simulink model "main_luenberger"  (R2016b)
settings: Solver=ode45  StartTime=0.0  StopTime=200  FixedStep=Par.Step_size  RelTol=1e-3
undefined symbols (not defined in the file or in its folder): now, Par
settings Model: Creator=Ørjan  LastModifiedBy=Ørjan
settings DataIOCC: InitialState=init  SaveState=on  ReturnWorkspaceOutputs=on  ReturnWorkspaceOutputsName=spidata
settings RTWCC: RTWCompilerOptimization=on
settings CodeAppCC: MaxIdLength=95

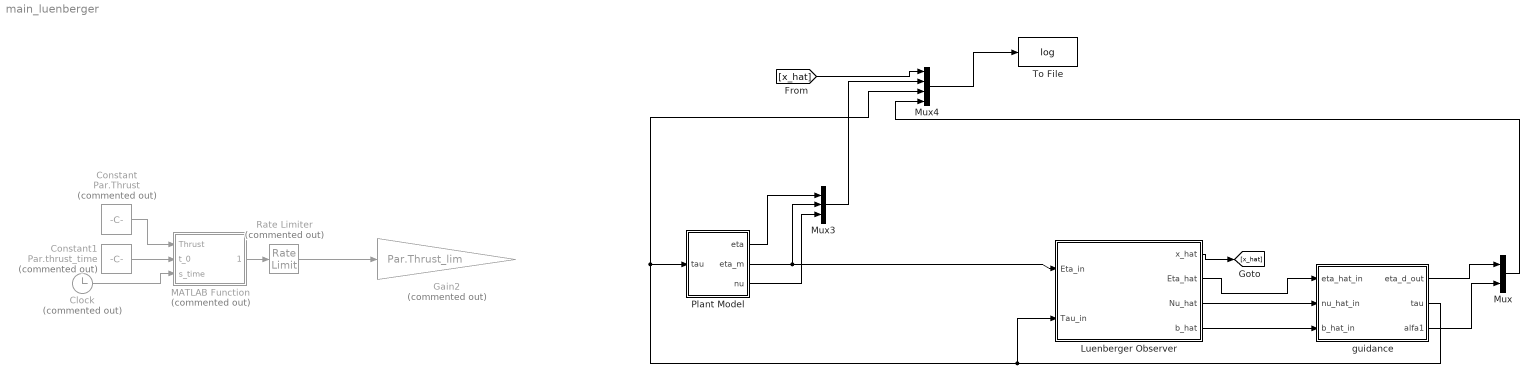
== system main_luenberger ==
  Clock : Clock  Commented=on
  Constant : Constant  Commented=on  Value=Par.Thrust  VectorParams1D=off
  Constant1 : Constant  Commented=on  Value=Par.thrust_time
  Gain2 : Gain  Commented=on  Gain=Par.Thrust_lim
  Luenberger Observer : Subsystem
  MATLAB Function : MATLAB Function  Commented=on  TreatAsAtomicUnit=on
  Mux : Mux  Inputs=2
  Mux3 : Mux  Inputs=3
  Mux4 : Mux
  Plant Model : Subsystem
  Rate Limiter : RateLimiter  Commented=on  RisingSlewLimit=5  FallingSlewLimit=-5  SampleTimeMode=inherited
  To File : ToFile  Filename=log  MatrixName=x  SampleTime=0.1
  guidance : Subsystem
  wires:
  Constant/1 -> MATLAB Function/1(Thrust)
  Clock/1 -> MATLAB Function/3(s_time)
  MATLAB Function/1(tau_norm) -> Rate Limiter/1
  Constant1/1 -> MATLAB Function/2(t_0)
  guidance/2(tau) -> Mux4/3, Plant Model/1(tau), Luenberger Observer/2(Tau_in)
  Rate Limiter/1 -> Gain2/1
  Plant Model/2(eta_m) -> Mux3/2, Luenberger Observer/1(Eta_in)
  Plant Model/1(eta) -> Mux3/1
  Plant Model/3(nu) -> Mux3/3
  Mux3/1 -> Mux4/2
  Mux4/1 -> To File/1
  [x_hat] -> Mux4/1
  Luenberger Observer/1("x_hat ") -> [x_hat]
  Luenberger Observer/3(Nu_hat) -> guidance/2(nu_hat_in)
  Luenberger Observer/2(Eta_hat) -> guidance/1("eta_hat_in ")
  Mux/1 -> Mux4/4
  Luenberger Observer/4(b_hat) -> guidance/3(b_hat_in)
  guidance/3(alfa1) -> Mux/2
  guidance/1(eta_d_out) -> Mux/1

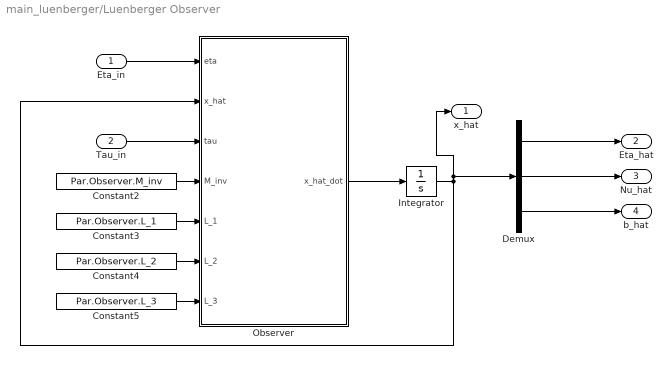
== system main_luenberger/Luenberger Observer ==
  Eta_in : Inport
  Tau_in : Inport  Port=2
  Constant2 : Constant  Value=Par.Observer.M_inv
  Constant3 : Constant  Value=Par.Observer.L_1
  Constant4 : Constant  Value=Par.Observer.L_2
  Constant5 : Constant  Value=Par.Observer.L_3
  Demux : Demux  Outputs=3
  Integrator : Integrator  InitialCondition=Par.Observer.x_0
  Observer : MATLAB Function  TreatAsAtomicUnit=on
  "x_hat " : Outport
  Eta_hat : Outport  Port=2  PortDimensions=[3, 1]
  Nu_hat : Outport  Port=3  PortDimensions=[3, 1]
  b_hat : Outport  Port=4  PortDimensions=[3, 1]
  wires:
  Constant3/1 -> Observer/5(L_1)
  Integrator/1 -> "x_hat "/1, Demux/1, Observer/2(x_hat)
  Demux/1 -> Eta_hat/1
  Demux/2 -> Nu_hat/1
  Observer/1(x_hat_dot) -> Integrator/1
  Constant2/1 -> Observer/4(M_inv)
  Eta_in/1 -> Observer/1(eta)
  Tau_in/1 -> Observer/3(tau)
  Constant4/1 -> Observer/6(L_2)
  Constant5/1 -> Observer/7(L_3)
  Demux/3 -> b_hat/1

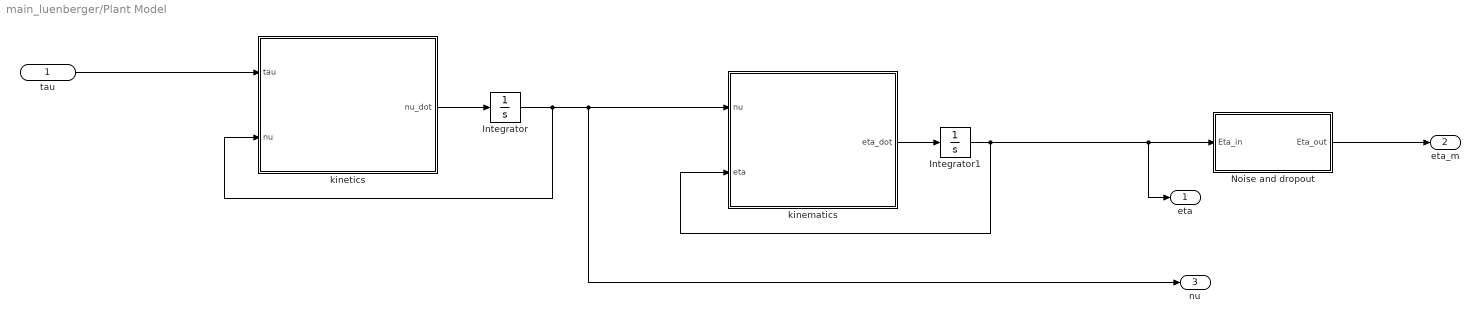
== system main_luenberger/Plant Model ==
  tau : Inport
  Integrator : Integrator  InitialCondition=[0 0 0]
  Integrator1 : Integrator  InitialCondition=[0 0 0]
  Noise and dropout : Subsystem
  kinematics : MATLAB Function  TreatAsAtomicUnit=on
  kinetics : MATLAB Function  TreatAsAtomicUnit=on
  eta : Outport
  eta_m : Outport  Port=2
  nu : Outport  Port=3
  wires:
  kinetics/1(nu_dot) -> Integrator/1
  kinematics/1(eta_dot) -> Integrator1/1
  Integrator/1 -> kinetics/2(nu), nu/1, kinematics/1(nu)
  Integrator1/1 -> eta/1, Noise and dropout/1(Eta_in), kinematics/2(eta)
  Noise and dropout/1(Eta_out) -> eta_m/1
  tau/1 -> kinetics/1(tau)

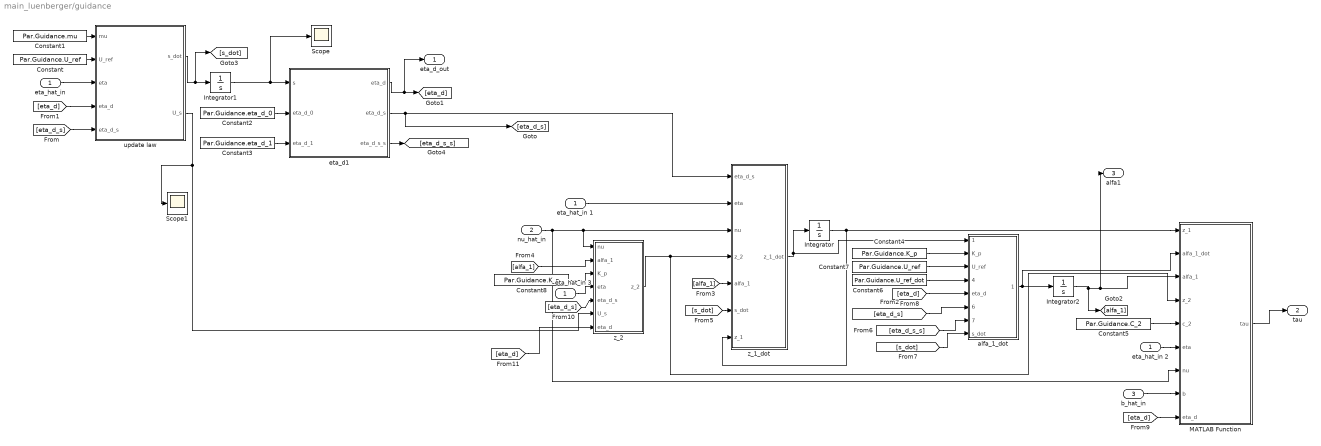
== system main_luenberger/guidance ==
  "eta_hat_in " : Inport
  nu_hat_in : Inport  Port=2
  b_hat_in : Inport  Port=3
  Constant : Constant  Value=Par.Guidance.U_ref
  Constant1 : Constant  Value=Par.Guidance.mu
  Constant2 : Constant  Value=Par.Guidance.eta_d_0
  Constant3 : Constant  Value=Par.Guidance.eta_d_1
  Constant4 : Constant  Value=Par.Guidance.K_p
  Constant5 : Constant  Value=Par.Guidance.C_2
  Constant6 : Constant  Value=Par.Guidance.U_ref_dot
  Constant7 : Constant  Value=Par.Guidance.U_ref
  Constant8 : Constant  Value=Par.Guidance.K_p
  Integrator : Integrator  InitialCondition=Par.Guidance.z_1_0
  Integrator1 : Integrator  InitialCondition=Par.Guidance.s_0
  Integrator2 : Integrator  InitialCondition=Par.Guidance.alfa_1_0
  MATLAB Function : MATLAB Function  TreatAsAtomicUnit=on
  Scope : Scope
  Scope1 : Scope
  alfa_1_dot : MATLAB Function  TreatAsAtomicUnit=on
  eta_d1 : MATLAB Function  TreatAsAtomicUnit=on
  eta_hat_in 1 : InportShadow
  eta_hat_in 2 : InportShadow
  eta_hat_in 3 : InportShadow
  update law : MATLAB Function  TreatAsAtomicUnit=on
  z_1_dot : MATLAB Function  TreatAsAtomicUnit=on
  z_2 : MATLAB Function  TreatAsAtomicUnit=on
  eta_d_out : Outport
  tau : Outport  Port=2
  alfa1 : Outport  Port=3
  wires:
  "eta_hat_in "/1 -> update law/3(eta)
  Constant/1 -> update law/2(U_ref)
  Constant1/1 -> update law/1(mu)
  update law/1(s_dot) -> [s_dot], Integrator1/1
  Integrator1/1 -> Scope/1, eta_d1/1(s)
  Constant2/1 -> eta_d1/2(eta_d_0)
  Constant3/1 -> eta_d1/3(eta_d_1)
  eta_d1/2(eta_d_s) -> [eta_d_s], z_1_dot/1(eta_d_s)
  [eta_d_s] -> update law/5(eta_d_s)
  eta_d1/1(eta_d) -> eta_d_out/1, [eta_d]
  [eta_d] -> update law/4(eta_d)
  nu_hat_in/1 -> z_2/1(nu), z_1_dot/3(nu), MATLAB Function/7(nu)
  eta_hat_in 1/1 -> z_1_dot/2(eta)
  z_1_dot/1(z_1_dot) -> Integrator/1, alfa_1_dot/1(z_1_dot)
  z_2/1(z_2) -> MATLAB Function/4(z_2), z_1_dot/4(z_2)
  Constant4/1 -> alfa_1_dot/2(K_p)
  [eta_d_s] -> alfa_1_dot/6(eta_d_s)
  alfa_1_dot/1(alfa_1_dot) -> MATLAB Function/2(alfa_1_dot), Integrator2/1
  Integrator/1 -> z_1_dot/7(z_1), MATLAB Function/1(z_1)
  Constant5/1 -> MATLAB Function/5(c_2)
  MATLAB Function/1(tau) -> tau/1
  Constant6/1 -> alfa_1_dot/4(U_ref_dot)
  Integrator2/1 -> alfa1/1, MATLAB Function/3(alfa_1), [alfa_1]
  [alfa_1] -> z_1_dot/5(alfa_1)
  [alfa_1] -> z_2/2(alfa_1)
  [s_dot] -> z_1_dot/6(s_dot)
  update law/2(U_s) -> z_2/6(U_s), Scope1/1
  b_hat_in/1 -> MATLAB Function/8(b)
  eta_hat_in 2/1 -> MATLAB Function/6(eta)
  [eta_d_s_s] -> alfa_1_dot/7(eta_d_s_s)
  [s_dot] -> alfa_1_dot/8(s_dot)
  eta_d1/3(eta_d_s_s) -> [eta_d_s_s]
  [eta_d] -> alfa_1_dot/5(eta_d)
  Constant7/1 -> alfa_1_dot/3(U_ref)
  [eta_d] -> MATLAB Function/9(eta_d)
  Constant8/1 -> z_2/3(K_p)
  eta_hat_in 3/1 -> z_2/4(eta)
  [eta_d_s] -> z_2/5(eta_d_s)
  [eta_d] -> z_2/7(eta_d)

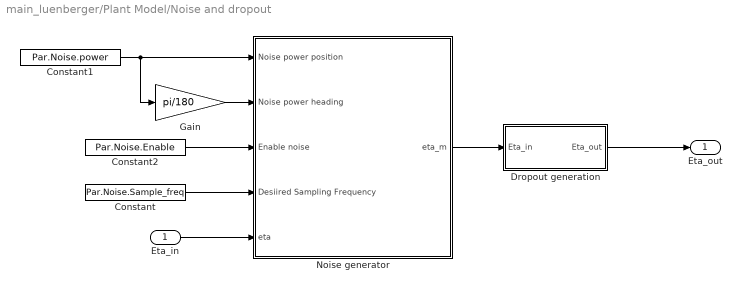
== system main_luenberger/Plant Model/Noise and dropout ==
  Eta_in : Inport
  Constant : Constant  Value=Par.Noise.Sample_freq
  Constant1 : Constant  Value=Par.Noise.power
  Constant2 : Constant  Value=Par.Noise.Enable
  Dropout generation : Subsystem
  Gain : Gain  Gain=pi/180
  Noise generator : Subsystem
  Eta_out : Outport
  wires:
  Constant2/1 -> Noise generator/3(Enable noise)
  Constant/1 -> Noise generator/4(Desiired Sampling Frequency)
  Gain/1 -> Noise generator/2(Noise power heading)
  Constant1/1 -> Noise generator/1(Noise power position), Gain/1
  Eta_in/1 -> Noise generator/5(eta)
  Noise generator/1(eta_m) -> Dropout generation/1(Eta_in)
  Dropout generation/1(Eta_out) -> Eta_out/1

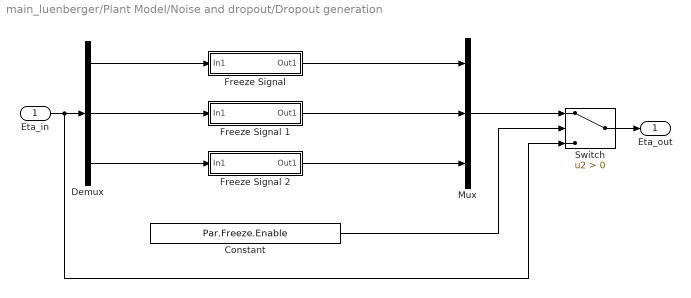
== system main_luenberger/Plant Model/Noise and dropout/Dropout generation ==
  Eta_in : Inport
  Constant : Constant  Value=Par.Freeze.Enable
  Demux : Demux  Outputs=3
  "Freeze Signal " : Subsystem
  Freeze Signal 1 : Subsystem
  Freeze Signal 2 : Subsystem
  Mux : Mux  Inputs=3
  Switch : Switch  Criteria=u2 > Threshold
  Eta_out : Outport
  wires:
  Switch/1 -> Eta_out/1
  Constant/1 -> Switch/2
  Freeze Signal 2/1(Out1) -> Mux/3
  Demux/3 -> Freeze Signal 2/1(In1)
  Demux/2 -> Freeze Signal 1/1(In1)
  Freeze Signal 1/1(Out1) -> Mux/2
  "Freeze Signal "/1(Out1) -> Mux/1
  Demux/1 -> "Freeze Signal "/1(In1)
  Mux/1 -> Switch/1
  Eta_in/1 -> Demux/1, Switch/3

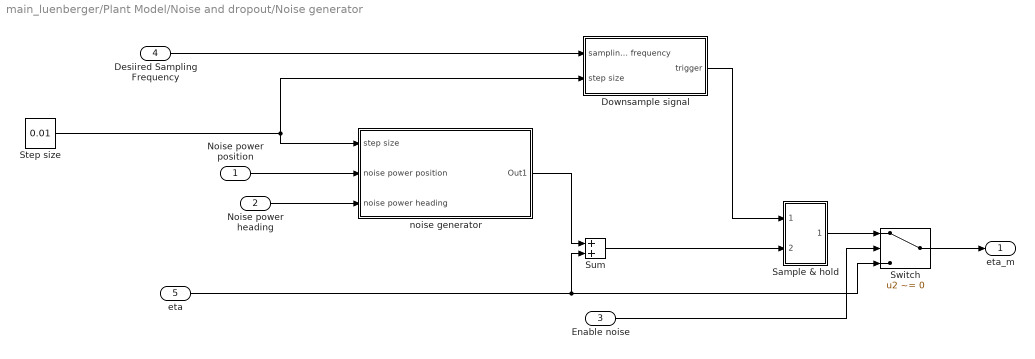
== system main_luenberger/Plant Model/Noise and dropout/Noise generator ==
  Noise power position : Inport
  Noise power heading : Inport  Port=2
  Enable noise : Inport  Port=3
  Desiired Sampling Frequency : Inport  Port=4
  eta : Inport  Port=5
  Downsample	signal : Subsystem
  Sample & hold : Subsystem
  Step size : Constant  Value=0.01
  Sum : Sum
  Switch : Switch  Criteria=u2 ~= 0
  noise generator : Subsystem
  eta_m : Outport
  wires:
  Switch/1 -> eta_m/1
  Enable noise/1 -> Switch/2
  noise generator/1(Out1) -> Sum/1
  Noise power heading/1 -> noise generator/3(noise power heading)
  Noise power position/1 -> noise generator/2(noise power position)
  Sample & hold/1(output) -> Switch/1
  Sum/1 -> Sample & hold/2(input)
  eta/1 -> Switch/3, Sum/2
  Desiired Sampling Frequency/1 -> Downsample	signal/1(sampling frequency)
  Downsample	signal/1(trigger) -> Sample & hold/1(trigger)
  Step size/1 -> noise generator/1(step size), Downsample	signal/2(step size)

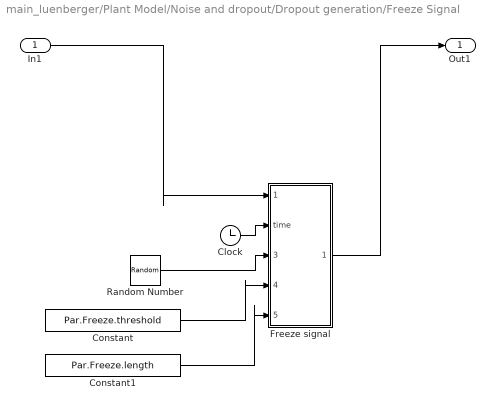
== system main_luenberger/Plant Model/Noise and dropout/Dropout generation/Freeze Signal  ==
  In1 : Inport
  Clock : Clock
  Constant : Constant  Value=Par.Freeze.threshold
  Constant1 : Constant  Value=Par.Freeze.length
  Freeze signal : MATLAB Function  TreatAsAtomicUnit=on
  Random Number : RandomNumber  Seed=ceil(abs(5*round(abs(now*1e6 - fix(now*1e6))*1e5)))  SampleTime=Par.Sample_time
  Out1 : Outport
  wires:
  Random Number/1 -> Freeze signal/3(random_value)
  Clock/1 -> Freeze signal/2(time)
  Constant/1 -> Freeze signal/4(threshold)
  Freeze signal/1(eta_out) -> Out1/1
  In1/1 -> Freeze signal/1(eta_in)
  Constant1/1 -> Freeze signal/5(length)

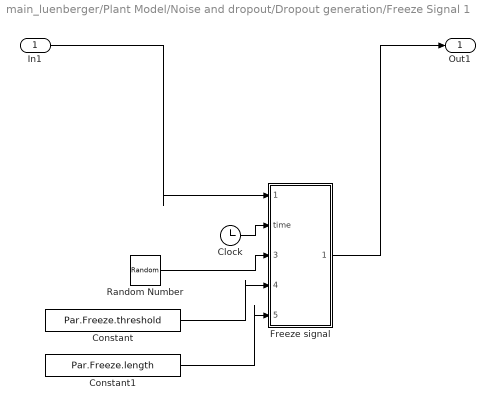
== system main_luenberger/Plant Model/Noise and dropout/Dropout generation/Freeze Signal 1 ==
  In1 : Inport
  Clock : Clock
  Constant : Constant  Value=Par.Freeze.threshold
  Constant1 : Constant  Value=Par.Freeze.length
  Freeze signal : MATLAB Function  TreatAsAtomicUnit=on
  Random Number : RandomNumber  Seed=ceil(abs(5*round(abs(now*1e6 - fix(now*1e6))*1e5)))  SampleTime=Par.Sample_time
  Out1 : Outport
  wires:
  Random Number/1 -> Freeze signal/3(random_value)
  Clock/1 -> Freeze signal/2(time)
  Constant/1 -> Freeze signal/4(threshold)
  Freeze signal/1(eta_out) -> Out1/1
  In1/1 -> Freeze signal/1(eta_in)
  Constant1/1 -> Freeze signal/5(length)

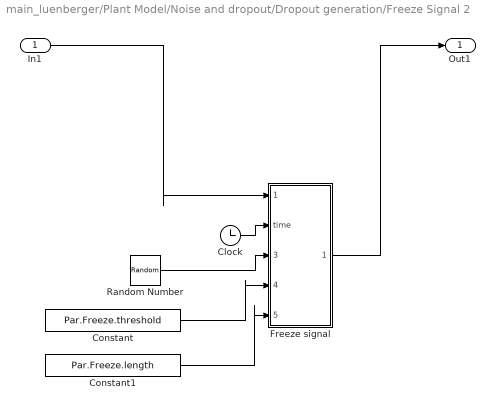
== system main_luenberger/Plant Model/Noise and dropout/Dropout generation/Freeze Signal 2 ==
  In1 : Inport
  Clock : Clock
  Constant : Constant  Value=Par.Freeze.threshold
  Constant1 : Constant  Value=Par.Freeze.length
  Freeze signal : MATLAB Function  TreatAsAtomicUnit=on
  Random Number : RandomNumber  Seed=ceil(abs(5*round(abs(now*1e6 - fix(now*1e6))*1e5)))  SampleTime=Par.Sample_time
  Out1 : Outport
  wires:
  Random Number/1 -> Freeze signal/3(random_value)
  Clock/1 -> Freeze signal/2(time)
  Constant/1 -> Freeze signal/4(threshold)
  Freeze signal/1(eta_out) -> Out1/1
  In1/1 -> Freeze signal/1(eta_in)
  Constant1/1 -> Freeze signal/5(length)

== system main_luenberger/Plant Model/Noise and dropout/Noise generator/Downsample	signal ==
  sampling frequency : Inport
  step size : Inport  Port=2
  MATLAB Function : MATLAB Function  TreatAsAtomicUnit=on
  counter : Memory
  trigger : Outport
  wires:
  MATLAB Function/1(count) -> trigger/1, counter/1
  counter/1 -> MATLAB Function/3(i)
  step size/1 -> MATLAB Function/2(h)
  sampling frequency/1 -> MATLAB Function/1(f)

== system main_luenberger/Plant Model/Noise and dropout/Noise generator/Sample & hold ==
  trigger : Inport
  input : Inport  Port=2
  Hold : Memory
  MATLAB Function1 : MATLAB Function  TreatAsAtomicUnit=on
  output : Outport
  wires:
  Hold/1 -> MATLAB Function1/3(hold)
  input/1 -> MATLAB Function1/2(input)
  trigger/1 -> MATLAB Function1/1(counter)
  MATLAB Function1/1(output) -> Hold/1, output/1

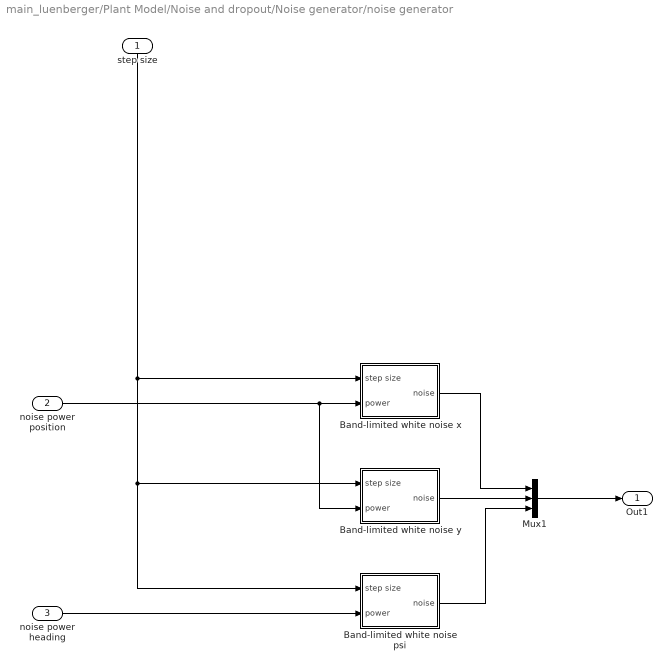
== system main_luenberger/Plant Model/Noise and dropout/Noise generator/noise generator ==
  step size : Inport
  noise power position : Inport  Port=2
  noise power heading : Inport  Port=3
  Band-limited white noise psi : Subsystem
  Band-limited white noise x : Subsystem
  Band-limited white noise y : Subsystem
  Mux1 : Mux  Inputs=3
  Out1 : Outport
  wires:
  noise power heading/1 -> Band-limited white noise psi/2(power)
  Band-limited white noise psi/1(noise) -> Mux1/3
  Band-limited white noise y/1(noise) -> Mux1/2
  Band-limited white noise x/1(noise) -> Mux1/1
  noise power position/1 -> Band-limited white noise x/2(power), Band-limited white noise y/2(power)
  step size/1 -> Band-limited white noise y/1(step size), Band-limited white noise psi/1(step size), Band-limited white noise x/1(step size)
  Mux1/1 -> Out1/1

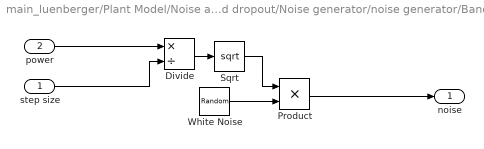
== system main_luenberger/Plant Model/Noise and dropout/Noise generator/noise generator/Band-limited white noise psi ==
  step size : Inport
  power : Inport  Port=2
  Divide : Product  Inputs=*/
  Product : Product
  Sqrt : Sqrt  SaturateOnIntegerOverflow=on
  White Noise : RandomNumber  DisableCoverage=on  Seed=9025  SampleTime=Par.Sample_time
  noise : Outport
  wires:
  power/1 -> Divide/1
  Sqrt/1 -> Product/1
  Divide/1 -> Sqrt/1
  step size/1 -> Divide/2
  Product/1 -> noise/1
  White Noise/1 -> Product/2

== system main_luenberger/Plant Model/Noise and dropout/Noise generator/noise generator/Band-limited white noise x ==
  step size : Inport
  power : Inport  Port=2
  Divide : Product  Inputs=*/
  Product : Product
  Sqrt : Sqrt  SaturateOnIntegerOverflow=on
  White Noise : RandomNumber  DisableCoverage=on  Seed=9024  SampleTime=Par.Sample_time
  noise : Outport
  wires:
  power/1 -> Divide/1
  Sqrt/1 -> Product/1
  Divide/1 -> Sqrt/1
  step size/1 -> Divide/2
  Product/1 -> noise/1
  White Noise/1 -> Product/2

== system main_luenberger/Plant Model/Noise and dropout/Noise generator/noise generator/Band-limited white noise y ==
  step size : Inport
  power : Inport  Port=2
  Divide : Product  Inputs=*/
  Product : Product
  Sqrt : Sqrt  SaturateOnIntegerOverflow=on
  White Noise : RandomNumber  DisableCoverage=on  Seed=123  SampleTime=Par.Sample_time
  noise : Outport
  wires:
  power/1 -> Divide/1
  Sqrt/1 -> Product/1
  Divide/1 -> Sqrt/1
  step size/1 -> Divide/2
  Product/1 -> noise/1
  White Noise/1 -> Product/2

== matlab function main_luenberger/Plant Model/kinematics ==
  data: nu input; eta_dot output; eta input
function eta_dot = CSE1_eta_dot(nu,eta)

psi = eta(3);

J = [cos(psi) -sin(psi) 0
     sin(psi) cos(psi)  0
     0        0         1];

eta_dot = J*nu;

== matlab function main_luenberger/Plant Model/kinetics ==
  data: tau input; nu_dot output; nu input
function nu_dot = CSE1_nu_dot(tau,nu)

u   = nu(1);
v   = nu(2);
r   = nu(3);

tau = [tau(1);tau(2);tau(3)];
%% MATRICES

m    = 14.79;   I_z  =  1.7600;   x_g = 0.0375;       % x_g  =  0.0460; % Table B.1


%% Added mass
X_ud  =     -2.0;											% Table B.1
					Y_vd =     -1.0;	N_vd =    -0.0;		% Table B.1 guestimate
					Y_rd =      -0.0;	N_rd =    -1.0;		% Table B.1

%% Total mass matrix
m_11 = m-X_ud;
m_22 = m-Y_vd;
m_23 = m*x_g-Y_rd;
m_32 = m*x_g-N_vd;
m_33 = I_z-N_rd;

M    = [m_11 0    0
        0    m_22 m_23
        0    m_32 m_33];
	
%% Damping coefficients
% Comments at the end of the lines indicate the old values used.
X_u		= -0.6555;		X_v		= 0;
X_uu 	= 0.3545;		X_vv	= -2.443;
X_uuu 	= -3.787;		X_vvv	= 0;

						Y_v		= -1.33; 			Y_r		= -7.250; % Y_r
						Y_vv	= -2.776;			Y_rr	= -3.450; % Y_rr
						Y_vvv	= -64.91;			Y_rrr	= 0;
						
						Y_rv	= -0.805;			Y_vr	= -0.845; % Y_rv, Y_vr

						N_v		= 0;				N_r		= -1.900; % N_r
						N_vv	= -0.2088;			N_rr	= -0.750; % N_rr
						N_vvv	= 0;				N_rrr	= 0;
						
						N_rv	= 0.130;			N_vr	= 0.080; % N_rv, N_vr

%% Correolis matrix
c_13 = -(m-Y_vd)*v-(m*x_g-Y_rd)*r;
c_23 = (m-X_ud)*u;
C    = [0     0     c_13
        0     0     c_23
        -c_13 -c_23 0   ];

%% Assembly of the damping matrix
d_11 = -X_u - X_uu*u - X_uuu*u^2;
d_22 = -Y_v - Y_vv*v - Y_vvv*v^2 - Y_rv*abs(r);
d_33 = -N_r - N_rr*abs(r) - N_rrr*r^2 - N_vr*abs(v); % using abs(r)

d_12 = -X_v - X_vv*v - X_vvv*v^2;
d_23 = -Y_r - Y_rr*abs(r) - Y_rrr*r^2 - Y_vr*abs(v);
d_32 = -N_v - N_vv*v - N_vvv*v^2 - N_rv*abs(r);

D    = [d_11 d_12 0
        0    d_22 d_23
        0    d_32 d_33];



%% CALCULATION
nu_dot = M\(tau-(C+D)*nu);

== matlab function main_luenberger/guidance/eta_d1 ==
  data: eta_d output size=3; s input; eta_d_0 input; eta_d_1 input; eta_d_s output; eta_d_s_s output
function [eta_d, eta_d_s, eta_d_s_s] = eta_d(s, eta_d_0, eta_d_1)
%% eta_d
x_d = (eta_d_1(1) - eta_d_0(1))*s + eta_d_0(1);
y_d = (eta_d_1(2) - eta_d_0(2))*s + eta_d_0(2);
psi_d = atan(y_d/x_d);
eta_d = [x_d; y_d; psi_d];

%% eta_d_s
x_d_s = eta_d_1(1) - eta_d_0(1);
y_d_s = eta_d_1(2) - eta_d_0(2);
psi_d_s = (y_d_s*eta_d(1) - eta_d(2)*x_d_s)/(eta_d(1)^2 + eta_d(2)^2);
eta_d_s = [x_d_s;y_d_s; psi_d_s];

%% eta_d_s_s
x_d_s_s = 0;
y_d_s_s = 0;
psi_d_s_s = (-2*(y_d_s*x_d - y_d*x_d_s)*(x_d*x_d_s + y_d*y_d_s))/(x_d^2+y_d^2)^2;
eta_d_s_s = [x_d_s_s;y_d_s_s;psi_d_s_s];
end

== matlab function main_luenberger/MATLAB Function ==
  data: tau_norm output; Thrust input; t_0 input; s_time input
function tau_norm = fcn(Thrust, t_0, s_time)
%coder.extrinsic('get_param');
tau_norm = zeros(3,1);
persistent i;
persistent tau;
if(isempty(i))
    i = 1;
end
if(isempty(tau))
    tau = [0; 0; 0];
end
if(s_time>t_0(i))
    tau(1) = Thrust(i, 1);
    tau(2) = Thrust(i, 2);
    tau(3) = Thrust(i, 3);
    if(i<size(Thrust, 1))
        i = i +1;
    end
end
tau_norm = tau;
end

== matlab function main_luenberger/guidance/update law ==
  data: mu input; s_dot output size=1; U_ref input; eta input; eta_d input; eta_d_s input; U_s output
function [s_dot, U_s] = s_dot(mu, U_ref, eta, eta_d, eta_d_s)
psi = eta(3);

R = [cos(psi) -sin(psi) 0; sin(psi) cos(psi) 0; 0 0 1];
z = R'*(eta-eta_d);
U_s = abs(U_ref)/norm(eta_d_s(1:2), 2);
V_1_s = -z'*R'*eta_d_s;
V_1_s = -(eta-eta_d)'*eta_d_s;
s_dot = U_s - (mu/norm(eta_d_s, 2))*V_1_s;
end

== matlab function main_luenberger/guidance/z_1_dot ==
  data: eta_d_s input; eta input; nu input; z_2 input; z_1_dot output size=3; alfa_1 input; s_dot input; z_1 input
function z_1_dot = z_1_dot(eta_d_s, eta, nu, z_2, alfa_1, s_dot, z_1)
psi = eta(3);
r = nu(3);
R = [cos(psi) -sin(psi) 0; sin(psi) cos(psi) 0; 0 0 1];
S = [0 -r 0; r 0 0; 0 0 0];
% z_1_dot = -S*z_1 + z_2 + alfa_1 - R'*eta_d_s*s_dot;
z_1_dot = -S*z_1 + nu - R'*eta_d_s*s_dot;
end

== matlab function main_luenberger/guidance/z_2 ==
  data: nu input; z_2 output; alfa_1 input size=3; K_p input; eta input; eta_d_s input; U_s input; eta_d input
function z_2= z_2(nu, alfa_1, K_p, eta, eta_d_s, U_s, eta_d)
psi = eta(3);
R = [cos(psi), -sin(psi), 0; sin(psi), cos(psi), 0; 0 0 1];
z_1 = R'*(eta-eta_d);
alfa1 = -K_p*z_1 + eta_d_s*U_s;
z_2 = nu - alfa_1;
end

== matlab function main_luenberger/guidance/alfa_1_dot ==
  data: z_1_dot input; K_p input; U_ref input; U_ref_dot input; eta_d input; eta_d_s input; alfa_1_dot output; eta_d_s_s input; s_dot input
function alfa_1_dot = alfa_1_dot(z_1_dot, K_p, U_ref, U_ref_dot, eta_d,eta_d_s, eta_d_s_s, s_dot)
% U_s_dot for straight line
U_s = U_ref/norm(eta_d(1:2), 2);
U_s_dot = U_ref_dot/norm(eta_d_s(1:2), 2);
% alfa_1_dot = -K_p*z_1_dot + eta_d_s*U_s_dot;
alfa_1_dot = -K_p*z_1_dot + eta_d_s*U_s_dot + eta_d_s_s*s_dot*U_s;
end

== matlab function main_luenberger/guidance/MATLAB Function ==
  data: z_1 input; alfa_1_dot input; alfa_1 input; tau output; z_2 input; c_2 input; eta input; nu input; b input; eta_d input
function tau = tau(z_1, alfa_1_dot, alfa_1, z_2, c_2, eta, nu, b, eta_d)
%% Damping coefficients
% Comments at the end of the lines indicate the old values used.
X_u		= -0.6555;		X_v		= 0;
X_uu 	= 0.3545;		X_vv	= -2.443;
X_uuu 	= -3.787;		X_vvv	= 0;

						Y_v		= -1.33; 			Y_r		= -7.250; % Y_r
						Y_vv	= -2.776;			Y_rr	= -3.450; % Y_rr
						Y_vvv	= -64.91;			Y_rrr	= 0;
						
						Y_rv	= -0.805;			Y_vr	= -0.845; % Y_rv, Y_vr

						N_v		= 0;				N_r		= -1.900; % N_r
						N_vv	= -0.2088;			N_rr	= -0.750; % N_rr
						N_vvv	= 0;				N_rrr	= 0;
						
						N_rv	= 0.130;			N_vr	= 0.080; % N_rv, N_vr
%% Assembly of the damping matrix
d_11 = -X_u - X_uu*abs(nu(1)) - X_uuu*nu(1)^2;
d_22 = -Y_v - Y_vv*abs(nu(2)) - Y_vvv*nu(2)^2 - Y_rv*abs(nu(3));
d_33 = -N_r - N_rr*abs(nu(3)) - N_rrr*nu(3)^2 - N_vr*abs(nu(2)); % using abs(r)

d_12 = -X_v - X_vv*abs(nu(2)) - X_vvv*nu(2)^2;
d_23 = -Y_r - Y_rr*abs(nu(3)) - Y_rrr*nu(3)^2 - Y_vr*abs(nu(2));
d_32 = -N_v - N_vv*abs(nu(2)) - N_vvv*nu(2)^2 - N_rv*abs(nu(3));

D    = [d_11 d_12 0
        0    d_22 d_23
        0    d_32 d_33];
%% Mass matrix
M = [16.79 0 0; 0 15.7900 0.5546; 0 0.5546 2.7600];
psi = eta(3);
R = [cos(psi) -sin(psi) 0; sin(psi) cos(psi) 0; 0 0 1];

%% tau
z_1 = R'*(eta-eta_d);
tau = -z_1 + D*nu + M*alfa_1_dot - c_2*z_2 -R'*b;
end

== matlab function main_luenberger/Plant Model/Noise and dropout/Dropout generation/Freeze Signal /Freeze signal ==
  data: eta_in input; eta_out output; time input; random_value input; threshold input; length input
function eta_out = fcn(eta_in, time, random_value, threshold, length)
persistent eta t_1;
if isempty(eta)
    eta = eta_in;
    t_1 = 0;
end

if random_value > threshold
    t_1 = time + length*(0.5*rand+0.5);
end
if time>=t_1
    eta = eta_in;
end

eta_out = eta;
end

== matlab function main_luenberger/Plant Model/Noise and dropout/Dropout generation/Freeze Signal 1/Freeze signal ==
  data: eta_in input; eta_out output; time input; random_value input; threshold input; length input
function eta_out = fcn(eta_in, time, random_value, threshold, length)
persistent eta t_1;
if isempty(eta)
    eta = eta_in;
    t_1 = 0;
end

if random_value > threshold
    t_1 = time + length*(0.5*rand+0.5);
end
if time>=t_1
    eta = eta_in;
end

eta_out = eta;
end

== matlab function main_luenberger/Plant Model/Noise and dropout/Dropout generation/Freeze Signal 2/Freeze signal ==
  data: eta_in input; eta_out output; time input; random_value input; threshold input; length input
function eta_out = fcn(eta_in, time, random_value, threshold, length)
persistent eta t_1;
if isempty(eta)
    eta = eta_in;
    t_1 = 0;
end

if random_value > threshold
    t_1 = time + length*(0.5*rand+0.5);
end
if time>=t_1
    eta = eta_in;
end

eta_out = eta;
end

== matlab function main_luenberger/Plant Model/Noise and dropout/Noise generator/Downsample	signal/MATLAB Function ==
  data: f input; h input; i input; count output
function count = fcn(f,h,i)
%#codegen
sampling_time = 1/f;
if (i+1)*h >= sampling_time
    count = 0;
else
    count = i+1;
end

== matlab function main_luenberger/Plant Model/Noise and dropout/Noise generator/Sample & hold/MATLAB Function1 ==
  data: counter input; input input; hold input; output output
function output = fcn(counter,input,hold)
%#codegen

if counter == 0
    output = input;
else
    output = hold;
end

== matlab function main_luenberger/Luenberger Observer/Observer ==
  data: eta input; x_hat_dot output; x_hat input; tau input; M_inv input; L_1 input; L_2 input; L_3 input
function x_hat_dot = fcn(eta, x_hat, tau, M_inv, L_1, L_2, L_3)
%#codegen

%Rotation matrix
R = [cos(eta(3)) -sin(eta(3)) 0; ...
    sin(eta(3)) cos(eta(3)) 0; ...
    0 0 1];
%% eta bar
eta_hat = x_hat(1:3);
eta_bar = eta - eta_hat;

nu_hat = x_hat(4:6);
b_hat = x_hat(7:9);
%% Damping coefficients
% Comments at the end of the lines indicate the old values used.
X_u		= -0.6555;		X_v		= 0;
X_uu 	= 0.3545;		X_vv	= -2.443;
X_uuu 	= -3.787;		X_vvv	= 0;

						Y_v		= -1.33; 			Y_r		= -7.250; % Y_r
						Y_vv	= -2.776;			Y_rr	= -3.450; % Y_rr
						Y_vvv	= -64.91;			Y_rrr	= 0;
						
						Y_rv	= -0.805;			Y_vr	= -0.845; % Y_rv, Y_vr

						N_v		= 0;				N_r		= -1.900; % N_r
						N_vv	= -0.2088;			N_rr	= -0.750; % N_rr
						N_vvv	= 0;				N_rrr	= 0;
						
						N_rv	= 0.130;			N_vr	= 0.080; % N_rv, N_vr
%% Assembly of the damping matrix
d_11 = -X_u - X_uu*abs(nu_hat(1)) - X_uuu*nu_hat(1)^2;
d_22 = -Y_v - Y_vv*abs(nu_hat(2)) - Y_vvv*nu_hat(2)^2 - Y_rv*abs(nu_hat(3));
d_33 = -N_r - N_rr*abs(nu_hat(3)) - N_rrr*nu_hat(3)^2 - N_vr*abs(nu_hat(2)); % using abs(r)

d_12 = -X_v - X_vv*abs(nu_hat(2)) - X_vvv*nu_hat(2)^2;
d_23 = -Y_r - Y_rr*abs(nu_hat(3)) - Y_rrr*nu_hat(3)^2 - Y_vr*abs(nu_hat(2));
d_32 = -N_v - N_vv*abs(nu_hat(2)) - N_vvv*nu_hat(2)^2 - N_rv*abs(nu_hat(3));

D    = [d_11 d_12 0
        0    d_22 d_23
        0    d_32 d_33];


%% x_dot equations
eta_hat_dot = R*nu_hat + L_1*eta_bar;
%nu_hat_dot = M_inv*(-D*nu_hat + R'*(b_hat + L_2*eta_bar) + tau);
nu_hat_dot = -M_inv*D*nu_hat + M_inv*R'*b_hat + M_inv*R'*L_2*eta_bar + M_inv*tau;
b_hat_dot = L_3*eta_bar;

x_hat_dot = [eta_hat_dot; nu_hat_dot; b_hat_dot];
end
